simulink model "mr_CoordinateTransformations"  (Simulink 7.5)
settings: Solver=FixedStepDiscrete  StartTime=0.0  StopTime=inf  FixedStep=SimSetup.baserate  RelTol=1e-3  SampleTimeConstraint=STIndependent
undefined symbols (not defined in the file): CentralBody, Time
libraries: CSA_Library x10
settings Model: Creator=salluda  LastModifiedBy=sufanmi
settings DataIOCC: ExternalInput=getinputstruct(op_HLV_Sim)  InitialState=getstatestruct(op_HLV_Sim)  SaveOutput=off  SignalLogging=off  SaveTime=off
settings OptimizationCC: InlineParams=on  EnforceIntegerDowncast=off  InitFltsAndDblsToZero=on  EfficientFloat2IntCast=on
settings DebuggingCC: SignalInfNanChecking=warning  SaveWithParameterizedLinksMsg=none  MultiTaskCondExecSysMsg=none  CheckMatrixSingularityMsg=warning  UnnecessaryDatatypeConvMsg=warning
settings HardwareCC: ProdHWDeviceType=32-bit Generic Real Time Simulator
settings ModelReferenceCC: UpdateModelReferenceTargets=IfOutOfDate
settings RTWCC: GenerateReport=on  ProcessScript=grt_make_rtw_hook  LaunchReport=on  TargetLang=C++  IncludeERTFirstTime=on
settings CodeAppCC: MaxIdLength=192
settings GRTTargetCC: TargetFcnLib=ansi_tfl_tmw.mat  UtilityFuncGeneration=Shared location  RTWCAPISignals=on  RTWCAPIParams=on

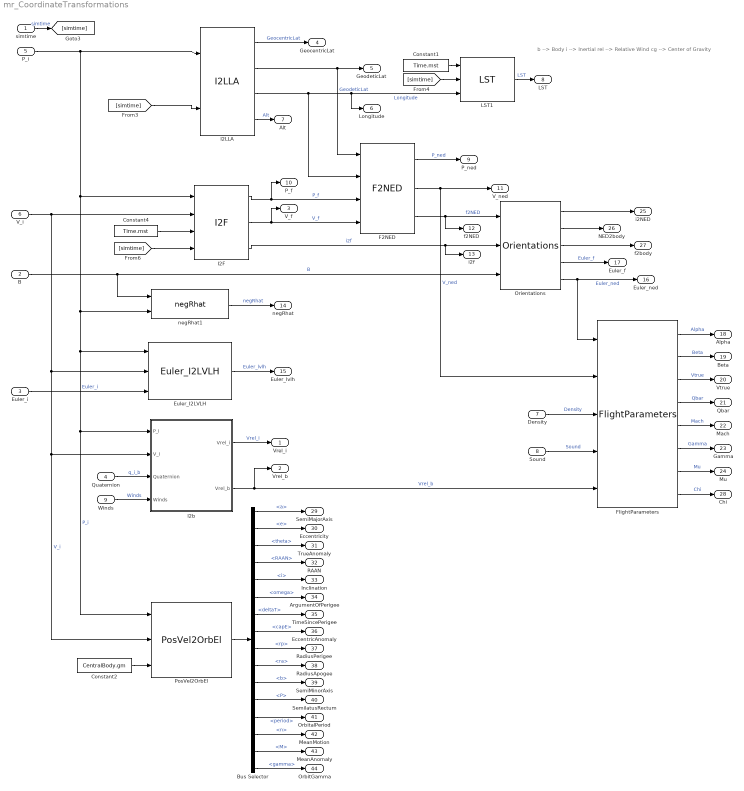
== system mr_CoordinateTransformations ==
  note: b   --> Body
      | i   --> Inertial
      | rel --> Relative Wind
      | cg  --> Center of Gravity
  simtime : Inport  PortDimensions=1  DataType=double  OutDataType=sfix(16)  OutScaling=2^0  OutDataTypeStr=double
  B : Inport  Port=2  PortDimensions=[3 3]  DataType=double  OutDataType=sfix(16)  OutScaling=2^0  OutDataTypeStr=double
  Euler_i : Inport  Port=3  PortDimensions=3  DataType=double  OutDataType=sfix(16)  OutScaling=2^0  OutDataTypeStr=double
  Quaternion : Inport  Port=4  PortDimensions=4  DataType=double  OutDataType=sfix(16)  OutScaling=2^0  OutDataTypeStr=double
  P_i : Inport  Port=5  PortDimensions=3  DataType=double  OutDataType=sfix(16)  OutScaling=2^0  OutDataTypeStr=double
  V_i : Inport  Port=6  PortDimensions=3  DataType=double  OutDataType=sfix(16)  OutScaling=2^0  OutDataTypeStr=double
  Density : Inport  Port=7  PortDimensions=1  DataType=double  OutDataType=sfix(16)  OutScaling=2^0  OutDataTypeStr=double
  Sound : Inport  Port=8  PortDimensions=1  DataType=double  OutDataType=sfix(16)  OutScaling=2^0  OutDataTypeStr=double
  Winds : Inport  Port=9  PortDimensions=3  DataType=double  OutDataType=sfix(16)  OutScaling=2^0  OutDataTypeStr=double
  Bus Selector : BusSelector  OutputSignals=a,e,theta,RAAN,i,omega,deltaT,capE,rp,ra,b,P,period,n,M,gamma
  Constant1 : Constant  Value=Time.mst  OutDataType=sfix(16)  OutScaling=2^0
  Constant2 : Constant  Value=CentralBody.gm  OutDataType=sfix(16)  OutScaling=2^0
  Constant4 : Constant  Value=Time.mst  OutDataType=sfix(16)  OutScaling=2^0
  Euler_I2LVLH : CSA_Library/CoordinateTransformations/Euler_I2LVLH  SystemSampleTime=-1
  F2NED : CSA_Library/CoordinateTransformations/F2NED  SystemSampleTime=-1
  FlightParameters : CSA_Library/FlightParameters/FlightParameters  SystemSampleTime=-1
  I2F : CSA_Library/CoordinateTransformations/I2F  SystemSampleTime=-1
  I2LLA : CSA_Library/CoordinateTransformations/I2LLA  SystemSampleTime=-1
  I2b : Subsystem
  LST1 : CSA_Library/CoordinateTransformations/LST  SystemSampleTime=-1
  Orientations : CSA_Library/CoordinateTransformations/Orientations  SystemSampleTime=-1
  PosVel2OrbEl : CSA_Library/OrbitalDynamics/PosVel2OrbEl  SystemSampleTime=-1
  negRhat1 : CSA_Library/CoordinateTransformations/negRhat  SystemSampleTime=-1
  Vrel_i : Outport  PortDimensions=3  DataType=double  OutDataType=sfix(16)  OutScaling=2^0  OutDataTypeStr=double
  Vrel_b : Outport  Port=2  PortDimensions=3  DataType=double  OutDataType=sfix(16)  OutScaling=2^0  OutDataTypeStr=double
  V_f : Outport  Port=3  PortDimensions=3  DataType=double  OutDataType=sfix(16)  OutScaling=2^0  OutDataTypeStr=double
  GeocentricLat : Outport  Port=4  PortDimensions=1  DataType=double  OutDataType=sfix(16)  OutScaling=2^0  OutDataTypeStr=double
  GeodeticLat : Outport  Port=5  PortDimensions=1  DataType=double  OutDataType=sfix(16)  OutScaling=2^0  OutDataTypeStr=double
  Longitude : Outport  Port=6  PortDimensions=1  DataType=double  OutDataType=sfix(16)  OutScaling=2^0  OutDataTypeStr=double
  Alt : Outport  Port=7  PortDimensions=1  DataType=double  OutDataType=sfix(16)  OutScaling=2^0  OutDataTypeStr=double
  LST : Outport  Port=8  PortDimensions=1  DataType=double  OutDataType=sfix(16)  OutScaling=2^0  OutDataTypeStr=double
  P_ned : Outport  Port=9  PortDimensions=3  DataType=double  OutDataType=sfix(16)  OutScaling=2^0  OutDataTypeStr=double
  P_f : Outport  Port=10  PortDimensions=3  DataType=double  OutDataType=sfix(16)  OutScaling=2^0  OutDataTypeStr=double
  V_ned : Outport  Port=11  PortDimensions=3  DataType=double  OutDataType=sfix(16)  OutScaling=2^0  OutDataTypeStr=double
  f2NED : Outport  Port=12  PortDimensions=[3 3]  DataType=double  OutDataType=sfix(16)  OutScaling=2^0  OutDataTypeStr=double
  i2f : Outport  Port=13  PortDimensions=[3 3]  DataType=double  OutDataType=sfix(16)  OutScaling=2^0  OutDataTypeStr=double
  negRhat : Outport  Port=14  PortDimensions=3  DataType=double  OutDataType=sfix(16)  OutScaling=2^0  OutDataTypeStr=double
  Euler_lvlh : Outport  Port=15  PortDimensions=3  DataType=double  OutDataType=sfix(16)  OutScaling=2^0  OutDataTypeStr=double
  Euler_ned : Outport  Port=16  PortDimensions=3  DataType=double  OutDataType=sfix(16)  OutScaling=2^0  OutDataTypeStr=double
  Euler_f : Outport  Port=17  PortDimensions=3  DataType=double  OutDataType=sfix(16)  OutScaling=2^0  OutDataTypeStr=double
  Alpha : Outport  Port=18  PortDimensions=1  DataType=double  OutDataType=sfix(16)  OutScaling=2^0  OutDataTypeStr=double
  Beta : Outport  Port=19  PortDimensions=1  DataType=double  OutDataType=sfix(16)  OutScaling=2^0  OutDataTypeStr=double
  Vtrue : Outport  Port=20  PortDimensions=1  DataType=double  OutDataType=sfix(16)  OutScaling=2^0  OutDataTypeStr=double
  Qbar : Outport  Port=21  PortDimensions=1  DataType=double  OutDataType=sfix(16)  OutScaling=2^0  OutDataTypeStr=double
  Mach : Outport  Port=22  PortDimensions=1  DataType=double  OutDataType=sfix(16)  OutScaling=2^0  OutDataTypeStr=double
  Gamma : Outport  Port=23  PortDimensions=1  DataType=double  OutDataType=sfix(16)  OutScaling=2^0  OutDataTypeStr=double
  Mu : Outport  Port=24  PortDimensions=1  DataType=double  OutDataType=sfix(16)  OutScaling=2^0  OutDataTypeStr=double
  i2NED : Outport  Port=25  PortDimensions=[3 3]  DataType=double  OutDataType=sfix(16)  OutScaling=2^0  OutDataTypeStr=double
  NED2body : Outport  Port=26  PortDimensions=[3 3]  DataType=double  OutDataType=sfix(16)  OutScaling=2^0  OutDataTypeStr=double
  f2body : Outport  Port=27  PortDimensions=[3 3]  DataType=double  OutDataType=sfix(16)  OutScaling=2^0  OutDataTypeStr=double
  Chi : Outport  Port=28  PortDimensions=1  DataType=double  OutDataType=sfix(16)  OutScaling=2^0  OutDataTypeStr=double
  SemiMajorAxis : Outport  Port=29  PortDimensions=1  OutDataType=sfix(16)  OutScaling=2^0
  Eccentricity : Outport  Port=30  PortDimensions=1  OutDataType=sfix(16)  OutScaling=2^0
  TrueAnomaly : Outport  Port=31  PortDimensions=1  OutDataType=sfix(16)  OutScaling=2^0
  RAAN : Outport  Port=32  PortDimensions=1  OutDataType=sfix(16)  OutScaling=2^0
  Inclination : Outport  Port=33  PortDimensions=1  OutDataType=sfix(16)  OutScaling=2^0
  ArgumentOfPerigee : Outport  Port=34  PortDimensions=1  OutDataType=sfix(16)  OutScaling=2^0
  TimeSincePerigee : Outport  Port=35  PortDimensions=1  OutDataType=sfix(16)  OutScaling=2^0
  EccentricAnomaly : Outport  Port=36  PortDimensions=1  OutDataType=sfix(16)  OutScaling=2^0
  RadiusPerigee : Outport  Port=37  PortDimensions=1  OutDataType=sfix(16)  OutScaling=2^0
  RadiusApogee : Outport  Port=38  PortDimensions=1  OutDataType=sfix(16)  OutScaling=2^0
  SemiMinorAxis : Outport  Port=39  PortDimensions=1  OutDataType=sfix(16)  OutScaling=2^0
  SemilatusRectum : Outport  Port=40  PortDimensions=1  OutDataType=sfix(16)  OutScaling=2^0
  OrbitalPeriod : Outport  Port=41  PortDimensions=1  OutDataType=sfix(16)  OutScaling=2^0
  MeanMotion : Outport  Port=42  PortDimensions=1  OutDataType=sfix(16)  OutScaling=2^0
  MeanAnomaly : Outport  Port=43  PortDimensions=1  OutDataType=sfix(16)  OutScaling=2^0
  OrbitGamma : Outport  Port=44  PortDimensions=1  OutDataType=sfix(16)  OutScaling=2^0
  wires:
  FlightParameters/7 -> Mu/1  "Mu"
  FlightParameters/5 -> Mach/1  "Mach"
  FlightParameters/4 -> Qbar/1  "Qbar"
  FlightParameters/3 -> Vtrue/1  "Vtrue"
  FlightParameters/2 -> Beta/1  "Beta"
  FlightParameters/1 -> Alpha/1  "Alpha"
  Orientations/5 -> Euler_ned/1, FlightParameters/1  "Euler_ned"
  Orientations/4 -> Euler_f/1  "Euler_f"
  Sound/1 -> FlightParameters/4  "Sound"
  Density/1 -> FlightParameters/3  "Density"
  Euler_I2LVLH/1 -> Euler_lvlh/1  "Euler_lvlh"
  F2NED/2 -> V_ned/1, FlightParameters/2  "V_ned"
  F2NED/1 -> P_ned/1  "P_ned"
  LST1/1 -> LST/1  "LST"
  I2LLA/4 -> Alt/1  "Alt"
  I2LLA/1 -> GeocentricLat/1  "GeocentricLat"
  I2b/1(Vrel_i) -> Vrel_i/1  "Vrel_i"
  I2b/2(Vrel_b) -> Vrel_b/1, FlightParameters/5  "Vrel_b"
  Quaternion/1 -> I2b/3(Quaternion)  "q_i_b"
  Winds/1 -> I2b/4(Winds)  "Winds"
  negRhat1/1 -> negRhat/1  "negRhat"
  Euler_i/1 -> Euler_I2LVLH/3  "Euler_i"
  B/1 -> negRhat1/1, Orientations/3  "B"
  F2NED/3 -> f2NED/1, Orientations/1  "f2NED"
  I2F/3 -> i2f/1, Orientations/2  "i2f"
  I2LLA/3 -> Longitude/1, LST1/3, F2NED/2  "Longitude"
  I2LLA/2 -> GeodeticLat/1, F2NED/1  "GeodeticLat"
  I2F/2 -> V_f/1, F2NED/4  "V_f"
  I2F/1 -> P_f/1, F2NED/3  "P_f"
  V_i/1 -> I2b/2(V_i), PosVel2OrbEl/2, Euler_I2LVLH/2, I2F/2  "V_i"
  [simtime] -> I2LLA/2
  P_i/1 -> I2b/1(P_i), PosVel2OrbEl/1, Euler_I2LVLH/1, negRhat1/2, I2F/1, I2LLA/1  "P_i"
  Constant4/1 -> I2F/3
  Constant1/1 -> LST1/1
  [simtime] -> LST1/2
  simtime/1 -> [simtime]  "simtime"
  [simtime] -> I2F/4
  Orientations/1 -> i2NED/1
  Orientations/2 -> NED2body/1
  Orientations/3 -> f2body/1
  FlightParameters/8 -> Chi/1  "Chi"
  FlightParameters/6 -> Gamma/1  "Gamma"
  Constant2/1 -> PosVel2OrbEl/3
  PosVel2OrbEl/1 -> Bus Selector/1
  Bus Selector/1 -> SemiMajorAxis/1  "<a>"
  Bus Selector/2 -> Eccentricity/1  "<e>"
  Bus Selector/3 -> TrueAnomaly/1  "<theta>"
  Bus Selector/4 -> RAAN/1  "<RAAN>"
  Bus Selector/5 -> Inclination/1  "<i>"
  Bus Selector/6 -> ArgumentOfPerigee/1  "<omega>"
  Bus Selector/7 -> TimeSincePerigee/1  "<deltaT>"
  Bus Selector/8 -> EccentricAnomaly/1  "<capE>"
  Bus Selector/9 -> RadiusPerigee/1  "<rp>"
  Bus Selector/10 -> RadiusApogee/1  "<ra>"
  Bus Selector/11 -> SemiMinorAxis/1  "<b>"
  Bus Selector/12 -> SemilatusRectum/1  "<P>"
  Bus Selector/13 -> OrbitalPeriod/1  "<period>"
  Bus Selector/14 -> MeanMotion/1  "<n>"
  Bus Selector/15 -> MeanAnomaly/1  "<M>"
  Bus Selector/16 -> OrbitGamma/1  "<gamma>"

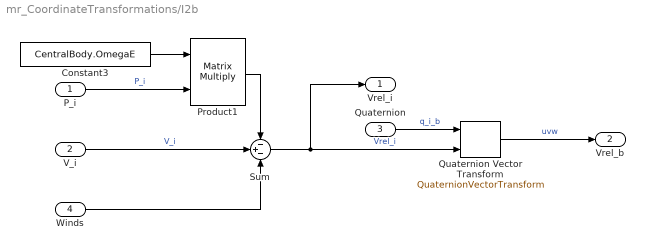
== system mr_CoordinateTransformations/I2b ==
  P_i : Inport  PortDimensions=3  OutDataType=sfix(16)  OutScaling=2^0
  V_i : Inport  Port=2  PortDimensions=3  OutDataType=sfix(16)  OutScaling=2^0
  Quaternion : Inport  Port=3  PortDimensions=4  OutDataType=sfix(16)  OutScaling=2^0
  Winds : Inport  Port=4  PortDimensions=3  OutDataType=sfix(16)  OutScaling=2^0
  Constant3 : Constant  Value=CentralBody.OmegaE  OutDataType=sfix(16)  OutScaling=2^0
  Product1 : Product  Multiplication=Matrix(*)  OutDataType=sfix(16)  OutScaling=2^0  SaturateOnIntegerOverflow=on  OutDataTypeStr=Inherit: Same as first input
  Quaternion Vector Transform : CSA_Library/CoordinateTransformations/QuaternionVectorTransform  SystemSampleTime=-1
  Sum : Sum  Inputs=-+-  OutDataType=sfix(16)  OutScaling=2^0
  Vrel_i : Outport  OutDataType=sfix(16)  OutScaling=2^0
  Vrel_b : Outport  Port=2  OutDataType=sfix(16)  OutScaling=2^0
  wires:
  Winds/1 -> Sum/3
  Sum/1 -> Quaternion Vector Transform/2, Vrel_i/1  "Vrel_i"
  P_i/1 -> Product1/2  "P_i"
  Quaternion/1 -> Quaternion Vector Transform/1  "q_i_b"
  Constant3/1 -> Product1/1
  V_i/1 -> Sum/2  "V_i"
  Quaternion Vector Transform/1 -> Vrel_b/1  "uvw"
  Product1/1 -> Sum/1
